simulink model "raspi_multicore_MPCtest_UD"  (R2021b)
settings: Solver=FixedStepDiscrete  StartTime=0.0  StopTime=600  FixedStep=0.005  RelTol=1e-3  EnableMultiTasking=on
InitFcn:
  | hardwareSetup;
values from neighbouring files (symbols this model uses):
  T_gait = 0.6    [MPCGen_OffsetFree.m]    (also in MPCGen_OffsetFree_UD.m = 0.65; MPCGen_OffsetFree_estDis.m; MPCcontrollerGen_OffsetFree.m = 0.7; MPCcontrollerGen_OffsetFree_UD.m = 0.65)
  Ts = 0.025    [MPCGen_OffsetFree.m]    (also in MPCGen_OffsetFree_UD.m = 0.02; MPCGen_OffsetFree_estDis.m = 0.03; MPCcontrollerGen_OffsetFree.m; MPCcontrollerGen_OffsetFree_UD.m = 0.02)
  Ts_DynSim = 0.005    [MPCGen_OffsetFree.m]    (also in MPCGen_OffsetFree_UD.m; MPCGen_OffsetFree_estDis.m = 0.006; MPCcontrollerGen_OffsetFree.m; MPCcontrollerGen_OffsetFree_UD.m)
libraries: PuppyLibrary x5, mpclib x1
settings Model: Creator=The MathWorks, Inc.  LastModifiedBy=kboxi
settings SolverCC: ConcurrentTasks=on  AlgebraicLoopSolver=TrustRegion  PositivePriorityOrder=on
settings OptimizationCC: EnhancedBackFolding=on  PassReuseOutputArgsThreshold=0  MaxStackSize=64  OptimizeBlockOrder=speed  DifferentSizesBufferReuse=on  OptimizationCustomize=off
settings DebuggingCC: ParameterTunabilityLossMsg=error  SFMachineParentedDataDiag=warning
settings HardwareCC: ProdBitPerPointer=32  ProdBitPerSizeT=32  ProdBitPerPtrDiffT=32  ProdLargestAtomicInteger=Long  ProdLargestAtomicFloat=Double  ProdWordSize=32  ProdLongLongMode=on  ProdHWDeviceType=ARM Compatible->ARM Cortex  UseEmbeddedCoderFeatures=off
settings RTWCC: Description=Embedded Coder  SystemTargetFile=ert.tlc  HardwareBoard=Raspberry Pi  TLCOptions="-aInlineSetEventsForThisBaseRateFcn=TLC_FALSE -aSuppressMultiTaskScheduler=TLC_FALSE  -aRateBasedStepFcn=0"  TemplateMakefile=ert_default_tmf  Toolchain=GNU GCC Embedded Linux  BuildConfiguration=Faster Runs
settings CodeAppCC: ForceParamTrailComments=on  OperatorAnnotations=on
settings ERTTargetCC: ERTCustomFileBanners=off  SupportContinuousTime=on  SupportNonInlinedSFcns=on  RemoveResetFunc=off  SupportVariableSizeSignals=on  ModelStepFunctionPrototypeControlCompliant=off

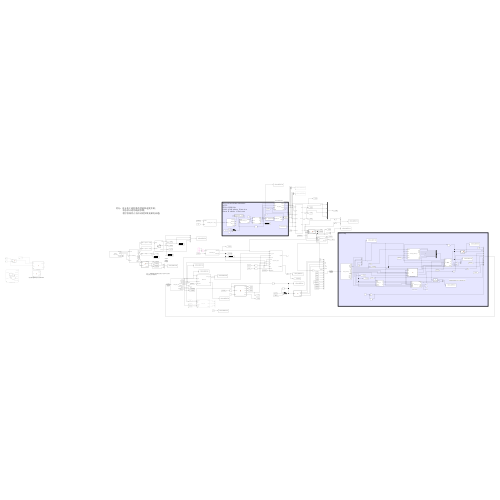
[thumbnail: Simulink's stored preview of the top-level diagram]
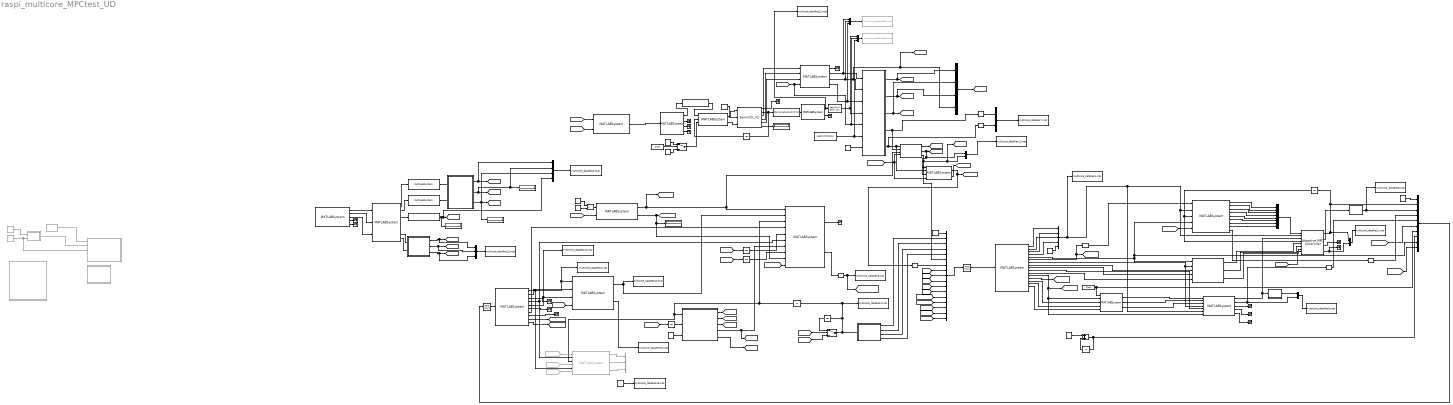
== system raspi_multicore_MPCtest_UD ==
  note: sitaErr=[0;0.005;0]
  note: Y 站立
      | X 踏步
      | B 急停
  note: 注意，从MPC输出的脚底位置是不包含2号电机与3号电机之间的偏移的。
  note: 待办：设计基于遥控器的使能和速度控制;
      | 状态估计处的地面参数;
      | 程序控制停止再启动的参数初始化问题；
  note: PendAll
  note: legState
  note: omega
  note: pCoM
  note: MPC Loop
  note: 考虑将LegState更换为touchInd
  note: 考虑将Inow替换为下位机实时计算
  note: Servo ctrl and State estimation
      | NOTE:
      | SPI fre: 2000 KHz
      | pCoM, vCoM, pArray_W are in m
      | pArray_B, pArray_L are in mm
  note: [0.007216;-0.002464;0.02254]
  note: vCoM
  note: RPY
  Adaptive MPC Controller1 : mpclib/Adaptive MPC Controller  SCDEnableBlockLinearizationSpecification=on  mpcobj=mpcPuppy  enable_value=0  updateMPCinCallerWorkspace=on  md_inport=off  mv_inport=on  uref_inport=off  return_cost=off  return_mvseq=off  return_qpstatus=on  return_xseq=on  return_state=off  return_ovseq=on  state_inport=off  isltv_plant=off  umin_inport=off  umax_inport=off  ymin_inport=off  ymax_inport=off  cc_inport=on  ywt_inport=off  uwt_inport=off  duwt_inport=off  rhoeps_inport=off  pm_inport=off  MaximumP=10  HorizonChoice=FixedHorizon  BlockDataType=double  SampleTimeInherited=on  switch_inport=on
  Add : Sum
  Bus Creator1 : BusCreator  Inputs=8
  Chart : Stateflow chart  TreatAsAtomicUnit=on
  Constant : Constant  Value=zeros(27,1)
  Constant{1,4,7..8} (4 alike) : Constant
  Constant15 : Constant  Commented=on  Value=0.001
  Constant2 : Constant  Value=9.8
  Constant20 : Constant  Commented=on
  Constant22 : Constant  Value=2*pi
  Constant23 : Constant  Value=T_gait
  Constant25 : Constant  Value=66
  Constant27 : Constant  Commented=on  Value=[0;0;0]
  Constant3 : Constant  Value=66
  Constant5 : Constant  Value=[0,0,0]
  Constant6 : Constant  Value=0
  Digital Clock : DigitalClock  SampleTime=Ts_DynSim
  Digital Clock2 : DigitalClock  SampleTime=Ts
  Display{,1..3,5} (5 alike) : Display
  Divide2 : Product  Inputs=*/
  From26 : From  Commented=on  GotoTag=LegState
  From27 : From  Commented=on  GotoTag=mpcSTOP
  From28 : From  Commented=on  GotoTag=pW
  JoyStick state machine : Stateflow chart  Commented=on  TreatAsAtomicUnit=on
  Leg Cor 2 Body Cor : PuppyLibrary/Leg Cor 2 Body Cor  SystemSampleTime=-1  VariantActivationTime=update diagram  Latency=0  AutoFrameSizeCalculation=off
  MATLAB Function : MATLAB Function  TreatAsAtomicUnit=on
  MATLAB Function1 : MATLAB Function  TreatAsAtomicUnit=on
  MATLAB Function2 : MATLAB Function  TreatAsAtomicUnit=on
  MATLAB Function3 : MATLAB Function  Commented=on  TreatAsAtomicUnit=on
  MATLAB Function4 : MATLAB Function  TreatAsAtomicUnit=on
  MATLAB Function5 : MATLAB Function  TreatAsAtomicUnit=on
  MATLAB Function6 : MATLAB Function  TreatAsAtomicUnit=on
  MATLAB System : MATLABSystem  System=JoystickRead  SampleTime=Ts_DynSim
      mask Type: JoystickRead
      mask Display:
      | disp(['Bluetooth' char(10) ' Joystick Reader']);
      | port_label('output',1,'EventNum');
      | port_label('output',2,'value');
      | port_label('output',3,'number');
      | port_label('output',4,'buttonState');
      | port_label('output',5,'axisState');
  MATLAB System1 : MATLABSystem  System=IMU_regulation  SimulateUsing=Code generation
      mask Type: IMU_regulation
      mask Display:
      | disp('IMU_regulation');
      | port_label('input',1,'acc');
      | port_label('input',2,'omega');
      | port_label('input',3,'rpy');
      | port_label('input',4,'OffEN');
      | port_label('output',1,'accOffnow');
      | port_label('output',2,'accL_W');
      | port_label('output',3,'omega_W');
      | port_label('output',4,'RPY');
  MATLAB System10 : MATLABSystem  System=UDP_decoder_raspi  Inorm=diag( [ 0.0078, 0.0275, 0.0328 ] )  m=3  hIni=0.19  lateral_width=0.097  sagetial_width=0.2108  roll_Off=0.037  SimulateUsing=Code generation
      mask Type: UDP_decoder_raspi
      mask Display:
      | disp('UDP_decoder_raspi');
      | port_label('input',1,'in');
      | port_label('output',1,'U');
      | port_label('output',2,'X_mpc');
      | port_label('output',3,'Inow');
      | port_label('output',4,'refP');
      | port_label('output',5,'SP_MPC');
      | port_label('output',6,'MPCtime');
      | port_label('output',7,'MPC_Count');
      | port_label('output',8,'EN');
      | port_label('output',9,'LegStateMPC');
      | port_label('output',10,'phiSlow');
  MATLAB System11 : MATLABSystem  System=PhaseOscillator_SG  SampleTime=Ts_DynSim  OffsetTime=0  TickTime=0.1  startPhase=0  SimulateUsing=Code generation
      mask Type: PhaseOscillator_SG
      mask Display:
      | disp('PhaseOscillator_SG');
      | port_label('input',1,'omega');
      | port_label('input',2,'EN');
      | port_label('output',1,'phaseNow');
      | port_label('output',2,'OscStopFlag');
  MATLAB System12 : MATLABSystem  System=footEndPos_protect  SimulateUsing=Code generation
      mask Type: footEndPos_protect
      mask Display:
      | disp('footEndPos_protect');
      | port_label('input',1,'PendAllL');
      | port_label('input',2,'ES');
      | port_label('output',1,'pArray_L');
  MATLAB System13 : MATLABSystem  System=FK  dt=0.005  SimulateUsing=Code generation
      mask Type: FK
      mask Display:
      | disp('FK');
      | port_label('input',1,'AngleArray');
      | port_label('output',1,'pArray_L');
      | port_label('output',2,'errFlag');
  MATLAB System14 : MATLABSystem  System=IK  LF_Off=[ 0; 0; 0 ]  RF_Off=[ 0; 0; 0 ]  LH_Off=[ 0; 0; 0 ]  RH_Off=[ 0; 0; 0 ]  SimulateUsing=Code generation
      mask Type: IK
      mask Display:
      | disp('IK');
      | port_label('input',1,'pArray_L');
      | port_label('output',1,'AngleArray');
      | port_label('output',2,'OffsetPArray');
      | port_label('output',3,'pArray_L_Out');
      | port_label('output',4,'errFlag');
  MATLAB System15 : MATLABSystem  System=message_decoder_PC  lateral_width=0.097  sagetial_width=0.2108  roll_Off=0.037  hIni=0.19  SimulateUsing=Code generation
      mask Type: message_decoder_PC
      mask Display:
      | disp('message_decoder_PC');
      | port_label('input',1,'in');
      | port_label('output',1,'pCoM');
      | port_label('output',2,'vCoM');
      | port_label('output',3,'RPYnew');
      | port_label('output',4,'OmegaW');
      | port_label('output',5,'SPLeg');
      | port_label('output',6,'SP');
      | port_label('output',7,'surVN');
      | port_label('output',8,'surV1');
      | port_label('output',9,'surV2');
      | port_label('output',10,'surP');
      | port_label('output',11,'headG');
      | port_label('output',12,'mpcStop');
      | port_label('output',13,'phi');
      | port_label('output',14,'vxPercent');
      | port_label('output',15,'vyPercent');
      | port_label('output',16,'wzPercent');
      | port_label('output',17,'estDis');
  MATLAB System16 : MATLABSystem  System=PosAssign_vel  cons_Vel=15  dt=Ts_DynSim  SimulateUsing=Code generation
      mask Type: PosAssign_vel
      mask Display:
      | disp('PosAssign_vel');
      | port_label('input',1,'PosDes');
      | port_label('input',2,'PosNow');
      | port_label('input',3,'EN');
      | port_label('output',1,'PosOut');
      | port_label('output',2,'setEN');
  MATLAB System17 : MATLABSystem  System=LegSequence_RT_v3  r0=[ 0; 0; 0.19 ]  theta0=[ 0; 0; 0 ]  dr0=[ 0; 0; 0 ]  omega0=[ 0; 0; 0 ]  lateral_width=0.097  sagetial_width=0.2108  roll_Off=0.037  m=3  kx=0.8  ky=0.8  kRz=0  T=T_gait  StepH=0.04  SampleTime=Ts_DynSim  OffsetTime=0  TickTime=0  startPhase=0  SimulateUsing=Code generation
      mask Type: LegSequence_RT_v3
      mask Display:
      | disp('LegSequence_RT_v3');
      | port_label('input',1,'phi');
      | port_label('input',2,'pArray_L_Adm');
      | port_label('input',3,'X_FB');
      | port_label('input',4,'MPC_Count');
      | port_label('input',5,'touchInd');
      | port_label('input',6,'ref');
      | port_label('input',7,'surP');
      | port_label('input',8,'zSur');
      | port_label('input',9,'OscStop');
      | port_label('input',10,'LegStateMPC');
      | port_label('output',1,'LegState');
      | port_label('output',2,'PendAllLocal');
  MATLAB System18 : MATLABSystem  System=groundAdaptionP1  lateral_width=0.097  sagetial_width=0.2108  roll_Off=0.037  SimulateUsing=Code generation
      mask Type: groundAdaptionP1
      mask Display:
      | disp('groundAdaptionP1');
      | port_label('input',1,'LegState');
      | port_label('input',2,'SP');
      | port_label('input',3,'touchInd');
      | port_label('input',4,'OscStop');
      | port_label('output',1,'pW');
      | port_label('output',2,'pW_LS');
  MATLAB System2 : MATLABSystem  System=AdmittanceCtr  lateral_width=0.097  sagetial_width=0.2108  roll_Off=0.037  hIni=0.19  m=3  ks1=25  ks2=25  ks3=25  bs1=0.1  bs2=0.1  bs3=0.1  dt=0.005  SimulateUsing=Code generation
      mask Type: AdmittanceCtr
      mask Display:
      | disp('AdmittanceCtr');
      | port_label('input',1,'U');
      | port_label('input',2,'X_mpc');
      | port_label('input',3,'SP_MPC');
      | port_label('input',4,'MPC_STOP');
      | port_label('output',1,'pArray_L_Adm');
      | port_label('output',2,'pLnor');
  MATLAB System20 : MATLABSystem  System=ssModelgen_OffsetFree_ID  Inorm=diag( [0.0046125 0.0230942 0.0253262] )  m=3  Ts=Ts  hIni=0.19  Ts_period=Ts_DynSim  SimulateUsing=Code generation
      mask Type: ssModelgen_OffsetFree_ID
      mask Display:
      | disp('ssModelgen_OffsetFree_ID');
      | port_label('input',1,'PendAll');
      | port_label('input',2,'YOld');
      | port_label('input',3,'UOld');
      | port_label('input',4,'SPLeg');
      | port_label('input',5,'disable');
      | port_label('output',1,'Anow');
      | port_label('output',2,'Bnow');
      | port_label('output',3,'Cnow');
      | port_label('output',4,'Dnow');
      | port_label('output',5,'X');
      | port_label('output',6,'U');
      | port_label('output',7,'Y');
      | port_label('output',8,'DX');
      | port_label('output',9,'Inow');
  MATLAB System3 : MATLABSystem  System=buttonDecoder_2  SimulateUsing=Code generation
      mask Type: buttonDecoder_2
      mask Display:
      | disp('buttonDecoder_2');
      | port_label('input',1,'Eventnum');
      | port_label('input',2,'value');
      | port_label('input',3,'number');
      | port_label('output',1,'X');
      | port_label('output',2,'Y');
      | port_label('output',3,'A');
      | port_label('output',4,'B');
      | port_label('output',5,'up');
      | port_label('output',6,'down');
      | port_label('output',7,'left');
      | port_label('output',8,'right');
      | port_label('output',9,'LAxis');
      | port_label('output',10,'RAxis');
  MATLAB System4 : MATLABSystem  System=edgeDetector  SimulateUsing=Code generation
      mask Type: edgeDetector
      mask Display:
      | disp('edgeDetector');
      | port_label('input',1,'dataNow');
      | port_label('output',1,'dataEdge');
  MATLAB System5 : MATLABSystem  Commented=on  System=Balance_QP  Inorm=diag([0.0046125 0.0230942 0.0253262])  m=3  Ts=Ts_DynSim  hIni=0.19  H=diag( [[1;1;5];[2;2;1];zeros(7,1)] )  SimulateUsing=Code generation
      mask Type: Balance_QP
      mask Display:
      | disp('Balance_QP');
      | port_label('input',1,'SP_MPC');
      | port_label('input',2,'xRef');
      | port_label('input',3,'xFB');
      | port_label('input',4,'LegState');
      | port_label('input',5,'U_MPC');
      | port_label('input',6,'disable');
      | port_label('output',1,'Xnew');
      | port_label('output',2,'Unew');
      | port_label('output',3,'exitflag');
  MATLAB System6 : MATLABSystem  System=ref_ctr  vxMax=0.2  vyMax=0.2  wzMax=0.8  SimulateUsing=Code generation
      mask Type: ref_ctr
      mask Display:
      | disp('ref_ctr');
      | port_label('input',1,'timeIn');
      | port_label('input',2,'disable');
      | port_label('input',3,'vxPercent');
      | port_label('input',4,'vyPercent');
      | port_label('input',5,'wzPercent');
      | port_label('output',1,'vx');
      | port_label('output',2,'vy');
      | port_label('output',3,'wz');
  MATLAB System7 : MATLABSystem  System=refTrajectory_v4  r0=[ 0; 0; 0.19 ]  theta0=[ 0; 0; 0 ]  dr0=[ 0; 0; 0 ]  omega0=[ 0; 0; 0 ]  desHeight=0.19  sitaErr_K=[0;0;0]  dt=Ts  numP=numP  SimulateUsing=Code generation
      mask Type: refTrajectory_v4
      mask Display:
      | disp('refTrajectory_v4');
      | port_label('input',1,'vxL');
      | port_label('input',2,'vyL');
      | port_label('input',3,'omegaZ');
      | port_label('input',4,'surVN');
      | port_label('input',5,'sura');
      | port_label('input',6,'X_FB');
      | port_label('input',7,'disable');
      | port_label('output',1,'refSeqOut');
      | port_label('output',2,'refP');
      | port_label('output',3,'refSeq');
      | port_label('output',4,'sitaErr');
      | port_label('output',5,'sitaNow');
  MATLAB System8 : MATLABSystem  System=ESgen  SimulateUsing=Code generation
      mask Type: ESgen
      mask Display:
      | disp('ESgen');
      | port_label('input',1,'trigger');
      | port_label('output',1,'ES');
  MATLAB System9 : MATLABSystem  System=edgeDetector  SimulateUsing=Code generation
      mask Type: edgeDetector
      mask Display:
      | disp('edgeDetector');
      | port_label('input',1,'dataNow');
      | port_label('output',1,'dataEdge');
  Mux : Mux
  Mux1 : Mux
  Mux{4,6..7,10} (4 alike) : Mux  Inputs=2
  Mux11 : Mux  Inputs=3
  Mux12 : Mux  Commented=on  Inputs=3
  Mux2 : Mux  Inputs=5
  Mux3 : Mux  Inputs=10
  Mux5 : Mux  Inputs=17
  Mux8 : Mux  Inputs=3
  Mux9 : Mux  Inputs=3
  Norminal_to_ServoAngle : PuppyLibrary/Norminal_to_ServoAngle  SystemSampleTime=-1  VariantActivationTime=update diagram  Latency=0  AutoFrameSizeCalculation=off
  Rate Transition : RateTransition  Deterministic=off  InitialCondition=zeros(67,1)  OutPortSampleTime=Ts_DynSim
  Rate Transition1 : RateTransition  Deterministic=off  InitialCondition=zeros(49,1)  OutPortSampleTime=Ts
  Reshape : Reshape
  Reshape1 : Reshape  OutputDimensionality=Customize  OutputDimensions=[3,4]
  Reshape2 : Reshape  OutputDimensionality=Customize  OutputDimensions=[4,1]
  Reshape3 : Reshape  OutputDimensionality=Customize  OutputDimensions=[12,1]
  Reshape4 : Reshape  OutputDimensionality=Customize  OutputDimensions=[13,1]
  Reshape5 : Reshape  OutputDimensionality=Customize  OutputDimensions=[9,1]
  Reshape6 : Reshape  OutputDimensionality=Customize  OutputDimensions=[12,1]
  ServoAngle_to_Norminal : PuppyLibrary/ServoAngle_to_Norminal  SystemSampleTime=-1  VariantActivationTime=update diagram  Latency=0  AutoFrameSizeCalculation=off
  ServoCtr_V2 : PuppyLibrary/ServoCtr_V2  SystemSampleTime=-1  VariantActivationTime=update diagram  Latency=0  AutoFrameSizeCalculation=off
  Subsystem : Subsystem
  Switch : Switch  Criteria=u2 > Threshold  Threshold=5
  Switch1 : Switch  Criteria=u2 > Threshold  Threshold=0.5
  Terminator{,1..16} (17 alike) : Terminator
  To File : ToFile  Filename=multicore_dataRec1.mat  MatrixName=rt_x_FB_slow
  To File1 : ToFile  Filename=multicore_dataRec2.mat  MatrixName=rt_mvOut_qpStatus_slow
  To File10 : ToFile  Commented=on  Filename=multicore_dataRecEstA.mat  MatrixName=rt_acc_omega_RPYOri
  To File11 : ToFile  Commented=on  Filename=multicore_dataRecEstB.mat  MatrixName=rt_pArrayB_EN_SW
  To File12 : ToFile  Filename=multicore_dataRec11.mat  MatrixName=rt_touchInd_LegState
  To File13 : ToFile  Filename=multicore_dataRec12.mat  MatrixName=rt_pLFKfast
  To File14 : ToFile  Filename=multicore_dataRec13.mat  MatrixName=rt_vxPercent_vyPercent_wzPercent
  To File15 : ToFile  Filename=multicore_dataRec14.mat  MatrixName=rt_spMPC_fast
  To File16 : ToFile  Filename=multicore_dataRec15.mat  MatrixName=rt_pLnor_fast
  To File17 : ToFile  Filename=multicore_dataRec16.mat  MatrixName=rt_qpXnew_qpUnew_qpExitFlag_fast
  To File2 : ToFile  Filename=multicore_dataRec3.mat  MatrixName=rt_mvOut_fast
  To File3 : ToFile  Filename=multicore_dataRec4.mat  MatrixName=rt_x_FB_fast
  To File4 : ToFile  Filename=multicore_dataRec5.mat  MatrixName=rt_PendAllLocal
  To File5 : ToFile  Filename=multicore_dataRec6.mat  MatrixName=rt_EstOff_OscEN_mpcSTOP_ES
  To File6 : ToFile  Filename=multicore_dataRec7.mat  MatrixName=rt_estSPLeg_estSP
  To File7 : ToFile  Filename=multicore_dataRec8.mat  MatrixName=rt_xMPCOut_slow
  To File8 : ToFile  Filename=multicore_dataRec9.mat  MatrixName=rt_refSeq2_refP_slow
  To File9 : ToFile  Filename=multicore_dataRec10.mat  MatrixName=rt_pArrayLAdm
  Unit Delay : UnitDelay  InitialCondition=zeros(12,1)  SampleTime=-1  HasFrameUpgradeWarning=on
  Unit Delay1 : UnitDelay  SampleTime=Ts  HasFrameUpgradeWarning=on
  Unit Delay2 : UnitDelay  InitialCondition=[0;0;7.5;0;0;7.5;0;0;7.5;0;0;7.5];  SampleTime=-1  HasFrameUpgradeWarning=on
  Unit Delay3 : UnitDelay  InitialCondition=[1,1,1,1]  SampleTime=-1  HasFrameUpgradeWarning=on
  Unit Delay4 : UnitDelay  InitialCondition=[0;0;0;0]  SampleTime=-1  HasFrameUpgradeWarning=on
  Unit Delay5 : UnitDelay  InitialCondition=[0.1075,0.1075,-0.1075,-0.1075;0.0750,-0.0750,0.0750,-0.0750;0,0,0,0];  SampleTime=-1  HasFrameUpgradeWarning=on
  Unit Delay6 : UnitDelay  InitialCondition=[0;0;0.19;zeros(9,1)]  SampleTime=-1  HasFrameUpgradeWarning=on
  Unit Delay7 : UnitDelay  InitialCondition=[0;0;0.19;zeros(9,1)]  SampleTime=-1  HasFrameUpgradeWarning=on
  getSwitchStatus : PuppyLibrary/getSwitchStatus  sampleTime=Ts_DynSim
  online Constraints1 : MATLAB Function  TreatAsAtomicUnit=on
  slopeGen1 : MATLAB Function  Commented=on  TreatAsAtomicUnit=on
  terrainSimulator1 : MATLAB Function  Commented=on  TreatAsAtomicUnit=on
  wires:
  MATLAB System10/1 -> To File2/1, MATLAB System2/1, MATLAB System5/5
  slopeGen1/1(sura) -> terrainSimulator1/2(surP2)
  [mpcSTOP] -> Mux5/13
  Reshape3/1 -> Mux5/7
  MATLAB Function2/4(surP) -> MATLAB System17/7, [surP]
  Constant22/1 -> Divide2/1
  Mux5/1 -> Rate Transition1/1
  Mux3/1 -> Rate Transition/1
  Rate Transition/1 -> MATLAB System10/1
  Constant23/1 -> Divide2/2
  MATLAB System10/2 -> MATLAB System2/2
  Constant25/1 -> Mux5/1
  Constant15/1 -> slopeGen1/1(slope)
  MATLAB System11/1 -> [phiFast], MATLAB Function4/3(phi), MATLAB System17/1  "phaseNow"
  Unit Delay6/1 -> MATLAB System17/3, MATLAB System5/3, MATLAB Function2/1(xFB)
  Constant27/1 -> terrainSimulator1/1(surP1)
  Divide2/1 -> MATLAB System11/1
  Constant20/1 -> terrainSimulator1/3(xBP), slopeGen1/2(startX)
  Unit Delay2/1 -> Adaptive MPC Controller1/4, MATLAB System20/3  "mvOld"
  MATLAB System15/5 -> online Constraints1/1(SPLeg), MATLAB System20/4, Mux3/9  "SPLeg"
  Digital Clock2/1 -> Mux3/7, MATLAB System6/1
  Adaptive MPC Controller1/3 -> Terminator7/1  "y_opt_state"
  Rate Transition1/1 -> MATLAB System15/1
  MATLAB System6/2 -> MATLAB System7/2
  MATLAB System20/1 -> Bus Creator1/1  "A"
  MATLAB System20/4 -> Bus Creator1/4  "D"
  MATLAB System15/3 -> Mux2/2  "sitaFB"
  Adaptive MPC Controller1/4 -> Terminator8/1, Mux6/2  "qp_status"
  MATLAB System7/4 -> Terminator5/1
  Constant3/1 -> Mux3/1
  online Constraints1/3(G) -> Adaptive MPC Controller1/7
  [DisSingal] -> Adaptive MPC Controller1/8
  MATLAB System15/11 -> online Constraints1/5(headG)
  MATLAB System7/2 -> Reshape4/1, Mux7/2  "refP"
  Reshape1/1 -> MATLAB System20/1  "PendAll"
  MATLAB System20/5 -> Bus Creator1/5  "X"
  Adaptive MPC Controller1/1 -> Mux6/1, Mux3/2, Unit Delay2/1  "mvOut"
  MATLAB System15/4 -> Mux2/4
  MATLAB System20/3 -> Bus Creator1/3  "C"
  MATLAB System15/8 -> online Constraints1/3(surV1)
  MATLAB System6/1 -> MATLAB System7/1  "vx"
  MATLAB System7/3 -> Terminator4/1
  Bus Creator1/1 -> Adaptive MPC Controller1/1
  MATLAB System20/8 -> Bus Creator1/8  "DX"
  MATLAB System20/2 -> Bus Creator1/2  "B"
  MATLAB System20/7 -> Bus Creator1/7  "Y"
  MATLAB Function1/1(y) -> To File7/1, Mux3/3  "X_mpc"
  MATLAB System15/7 -> MATLAB System7/4, online Constraints1/2(surVN)
  MATLAB System15/9 -> online Constraints1/4(surV2)
  MATLAB System6/3 -> MATLAB System7/3
  MATLAB System15/1 -> Mux2/1
  Reshape5/1 -> Mux3/4
  Mux2/1 -> To File/1, MATLAB System7/6, MATLAB System20/2, Adaptive MPC Controller1/2  "X_FB"
  online Constraints1/1(E) -> Adaptive MPC Controller1/5
  MATLAB System7/1 -> MATLAB Function6/1(u), Adaptive MPC Controller1/3
  MATLAB System7/5 -> Terminator6/1
  Constant2/1 -> Mux2/5
  online Constraints1/2(F) -> Adaptive MPC Controller1/6
  MATLAB System15/6 -> [SP_MPC], Reshape1/1  "SP"
  MATLAB System20/9 -> Reshape5/1  "Inow"
  MATLAB System15/10 -> MATLAB System7/5
  Reshape4/1 -> Mux3/5  "refP"
  MATLAB System15/12 -> [DisSingal], MATLAB System6/2, MATLAB System7/7
  MATLAB System15/2 -> Mux2/3
  MATLAB System20/6 -> Bus Creator1/6  "U"
  Adaptive MPC Controller1/2 -> MATLAB Function1/1(u)  "mpc_est_state"
  Reshape/1 -> [PendAllLocal], To File4/1
  MATLAB System1/4 -> Subsystem/3(RPYOri), Mux8/3  "RPY"
  Subsystem/4(SPLeg) -> MATLAB Function4/2(SPLeg), Reshape2/1  "SPLeg"
  MATLAB System1/2 -> Mux8/1, Subsystem/1(acc)  "acc"
  MATLAB System1/3 -> [omega], Mux/4, Subsystem/2(omega), Mux8/2  "omega"
  Leg Cor 2 Body Cor/1 -> Subsystem/4(pArray_B), Mux9/1
  ServoCtr_V2/5 -> MATLAB System1/3
  ServoCtr_V2/4 -> MATLAB System1/2
  ServoCtr_V2/6 -> Display5/1
  getSwitchStatus/1 -> Subsystem/6(SW), Mux9/3  "SW"
  ServoCtr_V2/1 -> Terminator10/1
  Unit Delay/1 -> MATLAB System16/2
  ServoCtr_V2/3 -> MATLAB System1/1
  MATLAB System12/1 -> MATLAB System14/1  "pArrayL_Des"
  Constant4/1 -> ServoCtr_V2/2
  Norminal_to_ServoAngle/1 -> MATLAB System16/1
  Constant7/1 -> Switch/3
  ServoAngle_to_Norminal/1 -> MATLAB System13/1
  MATLAB System13/2 -> Terminator1/1
  Constant6/1 -> Switch/1
  Subsystem/3(RPYnew) -> Mux/2, [RPY]  "RPYnew"
  Digital Clock/1 -> Switch/2
  Subsystem/2(vCoM) -> Mux/3, [vCoM]  "vCoM"
  Subsystem/1(pCoM) -> Mux/1, [pCoM]  "pCoM"
  Constant5/1 -> Subsystem/7(surArray)
  MATLAB System13/1 -> To File13/1, Leg Cor 2 Body Cor/1
  Switch/1 -> MATLAB System16/3
  MATLAB System16/1 -> ServoCtr_V2/1
  MATLAB System14/1 -> Norminal_to_ServoAngle/1
  MATLAB System14/3 -> Terminator3/1
  MATLAB System14/2 -> Terminator2/1
  MATLAB System14/4 -> Terminator9/1
  Subsystem/5(SP) -> MATLAB System18/2, MATLAB Function4/1(SP), Reshape6/1  "SP"
  ServoCtr_V2/2 -> Unit Delay/1, ServoAngle_to_Norminal/1
  MATLAB Function2/1(surVN) -> [surVN]
  MATLAB Function2/2(surV1) -> [surV1]
  MATLAB Function2/3(surV2) -> [surV2]
  MATLAB Function2/5(headG) -> [headG]
  [surVN] -> Mux5/8
  [surV1] -> Mux5/9
  [surV2] -> Mux5/10
  [surP] -> Mux5/11
  [headG] -> Mux5/12
  [touchInd] -> Unit Delay3/1
  MATLAB Function4/1(zSur) -> [zSur]
  [zSur] -> Unit Delay4/1
  [EstOff] -> Mux9/2, Subsystem/5(EN), MATLAB System1/4
  [PendAllLocal] -> MATLAB System12/1
  MATLAB System1/1 -> Terminator11/1
  MATLAB Function5/1(pCoM) -> Mux5/2
  MATLAB Function5/2(vCoM) -> Mux5/3
  MATLAB Function5/3(RPY) -> Mux5/4
  MATLAB Function5/4(Omega) -> Mux5/5
  Mux/1 -> [xFB]
  MATLAB System/1 -> MATLAB System3/1
  MATLAB System/2 -> MATLAB System3/2
  MATLAB System/3 -> MATLAB System3/3
  MATLAB System/4 -> Terminator12/1
  MATLAB System/5 -> Terminator13/1
  MATLAB System3/1 -> MATLAB System4/1
  MATLAB System4/1 -> Chart/1(stepEdge)
  Chart/1(estEN) -> [EstOff], Mux1/1
  Chart/2(oscEN) -> Mux1/2, Display2/1, [OscEN]
  [OscEN] -> MATLAB System11/2
  MATLAB System3/4 -> MATLAB System8/1
  MATLAB System8/1 -> Display1/1, Mux1/4, [ES]
  [ES] -> MATLAB System12/2
  MATLAB System11/2 -> Display3/1, MATLAB System17/9, [OscStopFlag]
  MATLAB Function4/2(touchInd) -> MATLAB System18/3, Mux10/1, [touchInd]
  [SP_MPC] -> Mux3/6
  MATLAB System16/2 -> ServoCtr_V2/3
  MATLAB System10/5 -> To File15/1, MATLAB System2/3
  [mpcSTOP] -> MATLAB System2/4
  MATLAB System2/1 -> MATLAB System17/2, To File9/1  "pArray_L_Adm"
  Constant1/1 -> Add/1
  Add/1 -> Unit Delay1/1, Mux3/8
  Unit Delay1/1 -> Add/2
  MATLAB System10/7 -> MATLAB System17/4
  Unit Delay3/1 -> MATLAB System17/5
  Unit Delay4/1 -> MATLAB System17/8
  MATLAB System10/4 -> MATLAB System5/2, MATLAB System17/6
  MATLAB System10/8 -> Terminator/1
  MATLAB System10/6 -> Terminator14/1
  MATLAB System10/3 -> Terminator15/1
  MATLAB System3/2 -> MATLAB System9/1
  MATLAB System9/1 -> Chart/2(standEdge)
  Chart/3(mpcSTOP) -> Mux1/3, Display/1, [mpcSTOP]  "mpcStop"
  [OscStopFlag] -> MATLAB System18/4, MATLAB Function4/4(OscStop)
  Mux1/1 -> To File5/1
  Switch1/1 -> Unit Delay7/1, To File3/1, Unit Delay6/1, MATLAB Function5/1(Xnow)
  [mpcSTOP] -> Switch1/2
  [xFB] -> Switch1/3  "Xnow"
  Unit Delay7/1 -> Switch1/1
  Mux4/1 -> To File6/1
  Reshape2/1 -> Mux4/1
  Reshape6/1 -> Mux4/2
  Mux6/1 -> To File1/1
  Mux7/1 -> To File8/1
  MATLAB Function6/1(y) -> Mux7/1  "refSeq2"
  Mux8/1 -> To File10/1
  Mux9/1 -> To File11/1
  MATLAB Function4/3(LegState) -> Mux5/6, MATLAB System18/1, [LegState], Mux10/2
  Mux10/1 -> To File12/1
  Constant8/1 -> MATLAB Function2/3(LOCK)
  MATLAB System18/2 -> [pW_LS]
  [pW_LS] -> Unit Delay5/1
  Unit Delay5/1 -> MATLAB Function2/2(PendAllLS)
  MATLAB System17/2 -> Reshape/1
  MATLAB System18/1 -> Reshape3/1, [pW]
  [DisSingal] -> MATLAB System20/5
  MATLAB System10/9 -> [LegStateMPC]
  [LegStateMPC] -> MATLAB System17/10
  [phiFast] -> Mux5/14
  MATLAB System15/13 -> [phiSlow]
  [phiSlow] -> Mux3/10
  MATLAB System10/10 -> [phiMPC]
  MATLAB System17/1 -> Terminator16/1
  MATLAB System3/9 -> MATLAB Function/1(leftaxis)
  MATLAB System3/10 -> MATLAB Function/2(rightaxis)
  MATLAB Function/1(vxPercent) -> Mux11/1, [vxPercent]
  MATLAB Function/2(vyPercent) -> Mux11/2, [vyPercent]
  MATLAB Function/3(wzPercent) -> Mux11/3, [wzPercent]
  [vxPercent] -> Mux5/15
  [vyPercent] -> Mux5/16
  [wzPercent] -> Mux5/17
  MATLAB System15/14 -> MATLAB System6/3
  MATLAB System15/15 -> MATLAB System6/4
  MATLAB System15/16 -> MATLAB System6/5
  Mux11/1 -> To File14/1
  MATLAB System2/2 -> To File16/1
  From26/1 -> MATLAB System5/4
  From27/1 -> MATLAB System5/6
  MATLAB System5/1 -> Mux12/1
  MATLAB System5/2 -> Mux12/2
  MATLAB System5/3 -> Mux12/3
  From28/1 -> MATLAB System5/1
  Constant/1 -> To File17/1

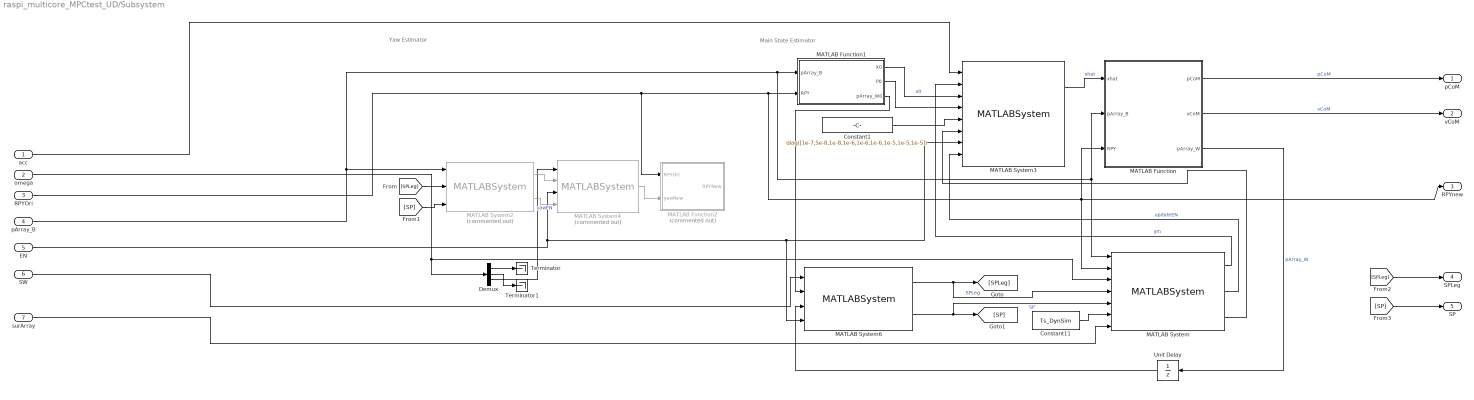
== system raspi_multicore_MPCtest_UD/Subsystem ==
  note: Yaw Estimator
  note: Main State Estimator
  acc : Inport
  omega : Inport  Port=2
  RPYOri : Inport  Port=3
  pArray_B : Inport  Port=4
  EN : Inport  Port=5
  SW : Inport  Port=6
  surArray : Inport  Port=7
  Constant1 : Constant  Value=diag([1e-7,5e-8,1e-8,1e-6,1e-6,1e-6,1e-5,1e-5,1e-5])
  Constant11 : Constant  Value=Ts_DynSim
  Demux : Demux  Outputs=3
  MATLAB Function : MATLAB Function  TreatAsAtomicUnit=on
  MATLAB Function1 : MATLAB Function  TreatAsAtomicUnit=on
  MATLAB Function2 : MATLAB Function  Commented=on  TreatAsAtomicUnit=on
  MATLAB System : MATLABSystem  System=estX_byJoint  SimulateUsing=Code generation
      mask Type: estX_byJoint
      mask Display:
      | disp('estX_byJoint');
      | port_label('input',1,'pArray_B');
      | port_label('input',2,'RPY');
      | port_label('input',3,'omegaB');
      | port_label('input',4,'SPLeg');
      | port_label('input',5,'SP');
      | port_label('input',6,'dt');
      | port_label('input',7,'surPara');
      | port_label('output',1,'ym');
      | port_label('output',2,'updateEN');
      | port_label('output',3,'KF_R');
  MATLAB System2 : MATLABSystem  Commented=on  System=yawEst_byJoint  dt=0.005  SimulateUsing=Code generation
      mask Type: yawEst_byJoint
      mask Display:
      | disp('yawEst_byJoint');
      | port_label('input',1,'pArray_B');
      | port_label('input',2,'SPLeg');
      | port_label('input',3,'SP');
      | port_label('output',1,'yawKine');
      | port_label('output',2,'updateEN');
  MATLAB System3 : MATLABSystem  System=KalmanFilter_DIY_Offrm  Ts=Ts_DynSim  SimulateUsing=Code generation
      mask Type: KalmanFilter_DIY_Offrm
      mask Display:
      | disp('KalmanFilter_DIY_Offrm');
      | port_label('input',1,'u');
      | port_label('input',2,'y');
      | port_label('input',3,'x0');
      | port_label('input',4,'p0');
      | port_label('input',5,'Q');
      | port_label('input',6,'R');
      | port_label('input',7,'Reset');
      | port_label('input',8,'updateEN');
      | port_label('output',1,'xhat');
      | port_label('output',2,'P');
  MATLAB System4 : MATLABSystem  Commented=on  System=KalmanFilter_DIY_yaw  A=1  B=Ts  C=1  G=1  x0=0  p0=1  Q=0.1  R=0.1  SimulateUsing=Code generation
      mask Type: KalmanFilter_DIY_yaw
      mask Display:
      | disp('KalmanFilter_DIY_yaw');
      | port_label('input',1,'u');
      | port_label('input',2,'y');
      | port_label('input',3,'Reset');
      | port_label('input',4,'updateEN');
      | port_label('output',1,'xhat');
  MATLAB System6 : MATLABSystem  System=LegStateIndicator  SimulateUsing=Code generation
      mask Type: LegStateIndicator
      mask Display:
      | disp('LegStateIndicator');
      | port_label('input',1,'SW');
      | port_label('input',2,'pArray_W0');
      | port_label('input',3,'pArray_W');
      | port_label('input',4,'reset');
      | port_label('output',1,'SPLeg');
      | port_label('output',2,'SP');
  Terminator : Terminator
  Terminator1 : Terminator
  Unit Delay : UnitDelay  InitialCondition=zeros(12,1)  SampleTime=-1  HasFrameUpgradeWarning=on
  pCoM : Outport
  vCoM : Outport  Port=2
  RPYnew : Outport  Port=3
  SPLeg : Outport  Port=4
  SP : Outport  Port=5
  wires:
  Demux/1 -> Terminator/1
  MATLAB System6/2 -> [SP], MATLAB System/5  "SP"
  MATLAB System/1 -> MATLAB System3/2  "ym"
  MATLAB System/2 -> MATLAB System3/8  "updateEN"
  Demux/3 -> MATLAB System4/1
  [SPLeg] -> MATLAB System2/2
  Constant1/1 -> MATLAB System3/5
  MATLAB System4/1 -> MATLAB Function2/2(yawNew)
  MATLAB System2/1 -> MATLAB System4/2
  MATLAB System3/1 -> MATLAB Function/1(xhat)  "xhat"
  pArray_B/1 -> MATLAB System2/1, MATLAB Function1/1(pArray_B), MATLAB Function/2(pArray_B), MATLAB System/1
  MATLAB Function1/1(X0) -> MATLAB System3/3  "x0"
  MATLAB Function/1(pCoM) -> pCoM/1  "pCoM"
  MATLAB System/3 -> MATLAB System3/6
  MATLAB System6/1 -> MATLAB System/4, [SPLeg]  "SPLeg"
  MATLAB Function1/3(pArray_W0) -> MATLAB System6/2
  Demux/2 -> Terminator1/1
  RPYOri/1 -> MATLAB Function2/1(RPYOri), MATLAB Function1/2(RPY), RPYnew/1, MATLAB Function/3(RPY), MATLAB System/2
  MATLAB Function/2(vCoM) -> vCoM/1  "vCoM"
  EN/1 -> MATLAB System4/3, MATLAB System3/7, MATLAB System6/4
  Constant11/1 -> MATLAB System/6
  MATLAB Function1/2(P0) -> MATLAB System3/4
  surArray/1 -> MATLAB System/7
  MATLAB Function/3(pArray_W) -> Unit Delay/1  "pArray_W"
  omega/1 -> Demux/1, MATLAB System/3
  MATLAB System2/2 -> MATLAB System4/4  "yawEN"
  [SP] -> MATLAB System2/3
  Unit Delay/1 -> MATLAB System6/3
  [SPLeg] -> SPLeg/1
  [SP] -> SP/1
  acc/1 -> MATLAB System3/1
  SW/1 -> MATLAB System6/1

== matlab function raspi_multicore_MPCtest_UD/Subsystem/MATLAB Function2 ==
  data: RPYOri input; RPYNew output size=[3 1]; yawNew input
function RPYNew = fcn(RPYOri,yawNew)
RPYNew=zeros(3,1);
RPYNew(1)=RPYOri(1);
RPYNew(2)=RPYOri(2);
RPYNew(3)=yawNew;

== matlab function raspi_multicore_MPCtest_UD/MATLAB Function2 ==
  data: xFB input; PendAllLS input; surVN output; surV1 output; surV2 output; surP output; headG output; LOCK input
function [surVN,surV1,surV2,surP,headG] = fcn(xFB,PendAllLS,LOCK)
W=[ones(4,1),PendAllLS(1,:)',PendAllLS(2,:)'];
a=pinv(W'*W)*W'*PendAllLS(3,:)';
theta=xFB(4:6);
surP=a;
if LOCK>0.5
    surP=[0;0;0];
    a=[0;0;0];
end

v1=[1;0;a(2)];
v2=[0;1;a(3)];
vT=cross(v1,v2);
vT=vT/norm(vT);

surVN=vT;
surV1=v1/norm(v1);
surV2=cross(surVN,surV1);

% if surVN'*[0;0;1]>cos(2/180*pi) % deadzone for terrain slope detection
%     surVN=[0;0;1];
%     surV1=[1;0;0];
%     surV2=[0;1;0];
%     surP=[0;0;0];
% end

Rx=[1,0,0;
    0,cos(theta(1)),-sin(theta(1));
    0,sin(theta(1)),cos(theta(1))];
Ry=[cos(theta(2)),0,sin(theta(2));
    0,1,0;
    -sin(theta(2)),0,cos(theta(2))];
Rz=[cos(theta(3)),-sin(theta(3)),0;
    sin(theta(3)),cos(theta(3)),0;
    0,0,1];
R=Rz*Ry*Rx;
headVL=[1;0;0];
headG=R*headVL;

== matlab function raspi_multicore_MPCtest_UD/MATLAB Function3 ==
  data: Xnow input; pCoM output; vCoM output; RPY output; Omega output
function [pCoM,vCoM,RPY,Omega] = fcn(Xnow)
pCoM=reshape(Xnow(1:3),3,1);
vCoM=reshape(Xnow(7:9),3,1);
RPY=reshape(Xnow(4:6),3,1);
Omega=reshape(Xnow(10:12),3,1);

== matlab function raspi_multicore_MPCtest_UD/slopeGen1 ==
  data: slope input; sura output; startX input
function sura = fcn(slope,startX)
slope=slope/180*pi;
surP1=[startX;1;0];
surP2=[startX;-1;0];
surP3=[startX+1;0;tan(slope)];
W=[1,surP1(1:2)';
    1,surP2(1:2)';
    1,surP3(1:2)'];

sura=(W'*W)\W'*[surP1(3);surP2(3);surP3(3);];

== matlab function raspi_multicore_MPCtest_UD/terrainSimulator1 ==
  data: surP1 input; touchInd output; surP2 input; xBP input; pendAll input; phi input; zSur output
function [touchInd,zSur] = fcn(surP1,surP2,xBP,pendAll,phi)
touchInd=zeros(4,1);
zSur=zeros(4,1);
LegState=[1;0;0;1];
s=phi/pi;
if phi>pi
    LegState=[0;1;1;0];
    s=s-1;
end
for i=1:1:4
    if LegState(i)<0.5 && s>0.2
        if pendAll(1,i)<xBP
            zSur(i)=[1;pendAll(1:2,i)]'*surP1;
        else
            zSur(i)=[1;pendAll(1:2,i)]'*surP2;
        end
        if pendAll(3,i)-zSur(i)<=0.001
            touchInd(i)=1;
        end
    end
end
end

== matlab function raspi_multicore_MPCtest_UD/MATLAB Function4 ==
  data: SP input; zSur output; SPLeg input; phi input; touchInd output; OscStop input; LegState output
function [zSur,touchInd,LegState] = fcn(SP,SPLeg,phi,OscStop)
zSur=reshape(SP(3,:),4,1);
LegState=[1;0;0;1];
touchInd=SPLeg;
s=phi/pi;
if phi>pi
    s=s-1;
    LegState=[0;1;1;0];
end
if abs(OscStop-1)<0.1
    LegState=[1;1;1;1];
end

for i=1:1:4
    if LegState(i)<0.5 && s>0.5
        if SPLeg(i)>0.5
            touchInd(i)=1;
        end
    end
end

== stateflow chart raspi_multicore_MPCtest_UD/Chart ==
  state StandBy
    entry:
    estEN=0;
    oscEN=0;
    mpcSTOP=1;
  state step_enable
    entry:
    estEN=0;
    oscEN=1;
    mpcSTOP=0;
  state MPC_enable_p1
    entry:
    estEN=1;
    oscEN=0;
    mpcSTOP=1;
  state MPC_enable_p2
    entry:
    estEN=0;
    oscEN=0;
    mpcSTOP=0;
  (default) -> StandBy
  StandBy -> MPC_enable_p1 : [standEdge==1]
  MPC_enable_p1 -> MPC_enable_p2 : [after(1,sec)]
  MPC_enable_p2 -> step_enable : [stepEdge==1]
  step_enable -> StandBy : [stepEdge==1]
  data: estEN output size=[1,1]; oscEN output size=[1,1]; stepEdge input size=[1,1]; mpcSTOP output size=[1,1]; standEdge input size=[1,1]

== matlab function raspi_multicore_MPCtest_UD/MATLAB Function6 ==
  data: u input; y output
function y = index_array(u)
y = u(2,1:13)';

== matlab function raspi_multicore_MPCtest_UD/MATLAB Function ==
  data: leftaxis input; vxPercent output; rightaxis input; vyPercent output; wzPercent output
function [vxPercent,vyPercent,wzPercent] = fcn(leftaxis,rightaxis)
vxPercent=leftaxis(1);
vyPercent=-leftaxis(2);
wzPercent=-rightaxis(2);

== stateflow chart raspi_multicore_MPCtest_UD/JoyStick state machine ==
  state TurnRight
    entry:
    TurnLeft=0;
    TurnRight=1;
  state Stop
    entry:
    PhaseOscEN=0;
  state Flat2Slope
    entry:
    TransCommand=1;
  state Forward
    entry:
    PhaseOscEN=1;
    ForwardAmp=1;
    AngleOffset=0;
    TurnLeft=0;
    TurnRight=0;
  state StandBy
    entry:
    PhaseOscEN=0;
    ForwardAmp=0;
    AngleOffset=0;
    TurnLeft=0;
    TurnRight=0;
    TransCommand=0;
  state ClearAngle
    entry:
    AngleOffset=1;
  state OnSpot
    entry:
    PhaseOscEN=1;
    ForwardAmp=0;
    AngleOffset=0;
    TurnLeft=0;
    TurnRight=0;
  state Continue
    entry:
    PhaseOscEN=1;
  state TurnLeft
    entry:
    TurnLeft=1;
    TurnRight=0;
  OnSpot -> TurnRight [order 2] : [JS_number==0 && JS_value>1000]
  TurnRight -> OnSpot [order 2] : [JS_number==0 && JS_value>1000 && ForwardAmp==0 && after(0.1,sec)]
  Forward -> TurnRight [order 1] : [JS_number==0 && JS_value>1000]
  TurnRight -> Forward [order 1] : [JS_number==0 && JS_value>1000 && ForwardAmp==1 && after(0.1,sec)]
  (default) -> StandBy
  Flat2Slope -> Stop : [JS_number==3 && JS_value==1]
  OnSpot -> Forward [order 1] : [JS_number==1 && JS_value<-1000]
  Forward -> Flat2Slope [order 2] : [JS_number==4 && JS_value==1]
  ClearAngle -> OnSpot : [after(1,sec)]
  StandBy -> ClearAngle : [JS_number==3 && JS_value==1]
  TurnLeft -> Forward [order 1] : [JS_number==0 && JS_value<-1000 && ForwardAmp==1 && after(0.1,sec)]
  Forward -> OnSpot [order 4] : [JS_number==1 && JS_value<-1000]
  Forward -> TurnLeft [order 3] : [JS_number==0 && JS_value<-1000]
  Stop -> Continue : [JS_number==3 && JS_value==1 && after(0.1,sec)]
  Continue -> Stop : [JS_number==3 && JS_value==1 && after(0.1,sec)]
  OnSpot -> StandBy [order 3] : [JS_number==3 && JS_value==1]
  OnSpot -> TurnLeft [order 4] : [JS_number==0 && JS_value<-1000]
  TurnLeft -> OnSpot [order 2] : [JS_number==0 && JS_value<-1000 && ForwardAmp==0 && after(0.1,sec)]
  data: JS_number input; JS_value input; TurnRight output; AngleOffset output; PhaseOscEN output; TurnLeft output; ForwardAmp output; TransCommand output

== matlab function raspi_multicore_MPCtest_UD/MATLAB Function1 ==
  data: u input; y output
function y = index_array(u)
y = u(2,1:13)';

== matlab function raspi_multicore_MPCtest_UD/Subsystem/MATLAB Function ==
  data: xhat input size=[9,1]; pCoM output size=[3,1]; vCoM output size=[3,1]; pArray_B input; RPY input; pArray_W output
function [pCoM,vCoM,pArray_W] = fcn(xhat,pArray_B,RPY)
% pB the CoM position in the world coordinate
% vB the CoM velocity
% Wpi the foot-end position in the world coordinate
pCoM=[xhat(1);xhat(2);xhat(3)];
vCoM=[xhat(4);xhat(5);xhat(6)];
Rz=[cos(RPY(3)),-sin(RPY(3)),0;
    sin(RPY(3)),cos(RPY(3)),0;
    0,0,1];
Ry=[cos(RPY(2)),0,sin(RPY(2));
    0,1,0;
    -sin(RPY(2)),0,cos(RPY(2))];
Rx=[1,0,0;
    0,cos(RPY(1)),-sin(RPY(1));
    0,sin(RPY(1)),cos(RPY(1))];
R=Rz*Ry*Rx;
pArray_B=reshape(pArray_B,3,4)/1000;
temp=R*pArray_B+pCoM*[1,1,1,1];
pArray_W=[temp(:,1);temp(:,2);temp(:,3);temp(:,4)];

== matlab function raspi_multicore_MPCtest_UD/online Constraints1 ==
  data: SPLeg input; E output; F output; G output; surVN input; surV1 input; surV2 input; headG input
function [E,F,G] = fcn(SPLeg,surVN,surV1,surV2,headG)
% surVN: unit norm vector of the surface
% surV1: unit actangular vector 1 of the surface
% surV2: unit actangular vector 2 of the surface
% headG: robot heading vector in world coordinate

%%%%%%%% set constraints %%%%%%%%%%
miu=0.6;
deltaFz=8; % w.r.t body coordinate
deltaFx=8; % w.r.t body coordinate
maxFz=60; % w.r.t. body coordinate

% friction cone----------------------
Eb2=zeros(8,12);
Gb2=zeros(8,1);
%Vb2=ones(8,1);
for i=1:1:4
    Eb2(i,3*i-2:3*i)=-miu*surVN+surV1;
    Eb2(i+4,3*i-2:3*i)=-miu*surVN-surV1;
end
Eb3=zeros(8,12);
Gb3=zeros(8,1);
%Vb3=ones(8,1);
for i=1:1:4
    Eb3(i,3*i-2:3*i)=-miu*surVN+surV2;
    Eb3(i+4,3*i-2:3*i)=-miu*surVN-surV2;
end
% payload balance--------------
surVhead=headG-headG'*surVN*surVN;
surVhead=surVhead/norm(surVhead);
Eb4=zeros(4,12);
Gb4=zeros(4,1);
%Vb4=ones(4,1);
Eb4(1,1:3)=surVhead;
Eb4(1,10:12)=-surVhead;
Eb4(2,1:3)=-surVhead;
Eb4(2,10:12)=surVhead;
Gb4(1)=deltaFx;
Gb4(2)=deltaFx;
Eb4(3,4:6)=surVhead;
Eb4(3,7:9)=-surVhead;
Eb4(4,4:6)=-surVhead;
Eb4(4,7:9)=surVhead;
Gb4(3)=deltaFx;
Gb4(4)=deltaFx;

Eb5=zeros(4,12);
Gb5=zeros(4,1);
%Vb5=ones(4,1);
Eb5(1,1:3)=surVN;
Eb5(1,10:12)=-surVN;
Eb5(2,1:3)=-surVN;
Eb5(2,10:12)=surVN;
Gb5(1)=deltaFz;
Gb5(2)=deltaFz;
Eb5(3,4:6)=surVN;
Eb5(3,7:9)=-surVN;
Eb5(4,4:6)=-surVN;
Eb5(4,7:9)=surVN;
Gb5(3)=deltaFz;
Gb5(4)=deltaFz;

% support force greater than zero, gait define----------
Eb1=zeros(8,12);
Gb1=zeros(8,1);
Vb1=ones(8,1)*0.1;
for i=1:1:4
    Eb1(i,3*i-2:3*i)=surVN;
    Eb1(i+4,3*i-2:3*i)=-surVN;
    Gb1(i)=maxFz;
    Gb1(i+4)=5;
end

for i=1:1:4
    if SPLeg(i)<0.5
        Gb1(i)=0;
        Gb1(i+4)=0;
    end
end

E=[Eb2;Eb3;Eb4;Eb5;Eb1];
F=zeros(32,13);
G=[Gb2;Gb3;Gb4;Gb5;Gb1];
%V=[Vb2;Vb3;Vb4;Vb5;Vb1];

% E=[Eb2;Eb3;Eb1];
% F=zeros(24,13);
% G=[Gb2;Gb3;Gb1];

%V=[Vb2;Vb3;Vb4;Vb5;Vb1];

== matlab function raspi_multicore_MPCtest_UD/MATLAB Function5 ==
  data: Xnow input; pCoM output; vCoM output; RPY output; Omega output
function [pCoM,vCoM,RPY,Omega] = fcn(Xnow)
pCoM=reshape(Xnow(1:3),3,1);
vCoM=reshape(Xnow(7:9),3,1);
RPY=reshape(Xnow(4:6),3,1);
Omega=reshape(Xnow(10:12),3,1);

== matlab function raspi_multicore_MPCtest_UD/Subsystem/MATLAB Function1 ==
  data: pArray_B input; RPY input; X0 output; P0 output; pArray_W0 output
function [X0,P0,pArray_W0]=fcn(pArray_B,RPY)
% NOTE: pArray_W0 is calculated without the value of yaw angle!!!
Ry=[cos(RPY(2)),0,sin(RPY(2));
    0,1,0;
    -sin(RPY(2)),0,cos(RPY(2))];
Rx=[1,0,0;
    0,cos(RPY(1)),-sin(RPY(1));
    0,sin(RPY(1)),cos(RPY(1))];
pArray_B=reshape(pArray_B,3,4)/1000;
pArray_float=Ry*Rx*pArray_B; % foot-end position in floating coordinate
zOff=-min(pArray_float(3,:));
temp=pArray_float+[0;0;zOff]*[1,1,1,1];
pCoM=[0;0;zOff];
vCoM=[0;0;0];
pArray_W0=[temp(:,1);temp(:,2);temp(:,3);temp(:,4)];
X0=[pCoM;vCoM;zeros(3,1)];
P0=eye(9)*10^-3;
